simulink model "MalhaContIA"  (R2015a)
settings: Solver=ode45  StartTime=0.0  StopTime=05  RelTol=1e-3
values from neighbouring files (symbols this model uses):
  A = [0 1; -3948 -1.26]    [Fuzzy_v3.m]
  Buw = [Bu, Bw]    [Fuzzy_v3.m]
  C = [12.5 0; -7896 -2.52]    [Fuzzy_v3.m]
  Duw = [Du, Dw]    [Fuzzy_v3.m]
  fis = addrule(fis, regras)    [Fuzzy_v3.m]
libraries: fuzblock x1
settings Model: Creator=ediva  LastModifiedBy=ediva

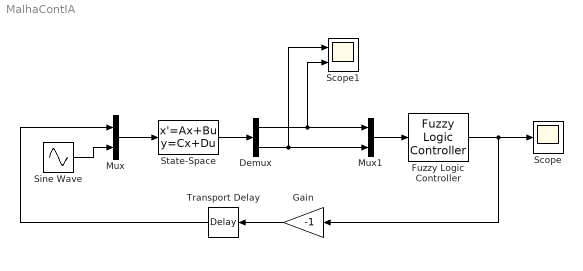
== system MalhaContIA ==
  Demux : Demux  Outputs=2
  Fuzzy Logic Controller : fuzblock/Fuzzy Logic  Controller  fis=[fis]
  Gain : Gain  Gain=-1
  Mux : Mux  Inputs=2
  Mux1 : Mux  Inputs=2
  Scope : Scope
  Scope1 : Scope  NumInputPorts=2
      settings: YMin=-17500~-30  YMax=17500~27.5
  Sine Wave : Sin  Amplitude=0.1  Frequency=62.83  SampleTime=0
  State-Space : StateSpace  A=A  B=Buw  C=C  D=Duw  X0=0
  Transport Delay : TransportDelay  DelayTime=0.0001
  wires:
  Mux/1 -> State-Space/1
  Fuzzy Logic Controller/1 -> Scope/1, Gain/1
  State-Space/1 -> Demux/1
  Mux1/1 -> Fuzzy Logic Controller/1
  Demux/1 -> Mux1/1, Scope1/2
  Demux/2 -> Scope1/1, Mux1/2
  Sine Wave/1 -> Mux/2
  Gain/1 -> Transport Delay/1
  Transport Delay/1 -> Mux/1
